simulink model "trackVehicleNewVer6b_Encoders_DR_GNC"  (R2018a)
settings: Solver=ode45  StartTime=0.0  StopTime=300  FixedStep=0.1  RelTol=1e-3  EnableMultiTasking=on
PreLoadFcn:
  | RTWConfigurationCB('preloadfcn', bdroot);
InitFcn:
  | parameterVehicle
  | parameterGNC
StartFcn:
  | start
StopFcn:
  | stop
  | 
  | myStopFcn2sim(xActEst,yActEst,X_array,Y_array,rp1,rp2)
values from neighbouring files (symbols this model uses):
  b = 0.29    [parameterVehicle.m]
  bDR = 1*b    [parameterGNC.m]
  dcArrayL = [-100 ... (first row only)    [parameterVehicle.m]
  dcArrayR = [-100 ... (first row only)    [parameterVehicle.m]
  eTick = 4300    [parameterVehicle.m]
  eTickDR = eTick    [parameterGNC.m]
  KP1 = 10    [parameterGNC.m]
  KP2 = 7    [parameterGNC.m]
  rl = 0.97*rNominal    (= 0.05982927699)    [parameterVehicle.m]
  rNominalDR = rNominal    [parameterGNC.m]
  rp1 = 0.4    [parameterGNC.m]
  rp2 = bDR    [parameterGNC.m]
  rr = 1.00*rNominal    (= 0.061679667)    [parameterVehicle.m]
  Tau1 = 0.001    [parameterGNC.m]
  Tau2 = 0.01    [parameterGNC.m]
  TauEncoderDR = 0.001    [parameterGNC.m]
  thetaIC = 180*(pi/180)    (= 3.14159265359)    [parameterVehicle.m]    (also in start.m = 1*double(c.Data) * pi/180)
  Tsample = 1/10    (= 0.1)    [parameterGNC.m]
  TsampleEncoder = 1/10    (= 0.1)    [parameterVehicle.m]
  TsampleEncoderDR = TsampleEncoder    [parameterGNC.m]
  Vcom = 3*VmaxDR/4    [parameterGNC.m]
  wArrayL = [-1.622403101 ... (first row only)    [parameterVehicle.m]
  wArrayR = [-1.288449612 ... (first row only)    [parameterVehicle.m]
  X_array = [-2 -2 0 0]    [parameterGNC.m]
  xIC = 0    [parameterVehicle.m]
  Y_array = [0 -3 -3 0]    [parameterGNC.m]
  yIC = 0    [parameterVehicle.m]
undefined symbols (not defined in the file or in its folder): DiscIntNeverNeededParam, Earth, WGS84
libraries: simulink x18, robotlib x14, simulink_extras x1, aerolibtransform2 x1
(part 2 of 2)

== matlab function trackVehicleNewVer6b_Encoders_DR_GNC/GNC/Navigation (DeadReckoning)/Kalman Filter ==
  data: xGPS input; yGPS input; thetaCompass input; VGPS input; omegaGyro input; wL input; wR input; st output; Tsample parameter; rNominalDR parameter; bDR parameter; covv output
function [st,covv] =  ExtKalman(xGPS,yGPS,thetaCompass,VGPS,omegaGyro,wL,wR,Tsample,rNominalDR,bDR)
%#codegen


meas=[xGPS;yGPS;thetaCompass;VGPS;omegaGyro];
persistent P xhat 
if isempty(P)
   % First time through the code so do some initialization
   xhat = zeros(5,1);
   P = zeros(5,5);
 end 
   Q = diag([.01 .01 .7 .01 .5]);
   R = 130*diag([1 1 1 1 1]);

% Calculate the Jacobians for the state and measurement equations
F = [1 0  -Tsample*xhat(4)*sin(xhat(3)) Tsample*cos(xhat(3)) 0 ;
     0 1   Tsample*xhat(4)*cos(xhat(3)) Tsample*sin(xhat(3)) 0 ;
     0 0            1                 0           Tsample ;
     0 0            0                 0            0 ;
     0 0            0                 0            0 ];
H = [0 0 0 0 0;
     0 0 0 0 0;
     0 0 1 0 0;
     0 0 0 1 0;
     0 0 0 0 1];
% Propogate  the state and covariance matrices
xhat = [...
    xhat(1) + Tsample*xhat(4)*cos(xhat(3));
    xhat(2) + Tsample*xhat(4)*sin(xhat(3));
    xhat(3) + Tsample* xhat(5);
    rNominalDR*(wL+wR)/2;
    rNominalDR*(wL-wR)/bDR];


P = F*P*F' + Q;
% Calculate the Kalman gain
K = P*H'/(H*P*H' + R);
% Calculate the measurement residual
yhat = H*xhat;
resid = meas - yhat;
% Update the state and covariance estimates
xhat = xhat + K*resid;
P = (eye(size(K,1))-K*H)*P;
% Post the results
st = xhat;
covv = P;

== matlab function trackVehicleNewVer6b_Encoders_DR_GNC/GNC/Navigation (DeadReckoning)/Sensor Suite/MATLAB Function ==
  data: x input; r output; y input
function r = ResultantVector(x, y)

r = sqrt(x^2 + y^2);

== matlab function trackVehicleNewVer6b_Encoders_DR_GNC/GNC/Navigation (DeadReckoning)/Sensor Suite/MATLAB Function1 ==
  data: x input; r output; y input
function r = ResultantVector(x, y)

r = sqrt(x^2 + y^2);

== matlab function trackVehicleNewVer6b_Encoders_DR_GNC/SendDutyToVehicle/MATLAB Function ==
  data: DutyCycle input; PWM output
function PWM = fcn(DutyCycle)
  

        PWM = int16(DutyCycle/100 * 255);
    end

== matlab function trackVehicleNewVer6b_Encoders_DR_GNC/SendDutyToVehicle/MATLAB Function4 ==
  data: DutyCycle input; PWM output
function PWM = fcn(DutyCycle)

    PWM = int16(DutyCycle/100 * 255);
